simulink model "Outer_Tensor_Stream_Ex1"  (R2025a)
settings: Solver=VariableStepAuto  StartTime=0.0  StopTime=1024  RelTol=1e-3
undefined symbols (not defined in the file): Correlation_ValidMode, DUT, L, vsva1596, xcvc1702
libraries: aieUtilities x8, aieDSP x1, vmcUtilities x1
settings Model: Creator=sdegala  LastModifiedBy=sdegala

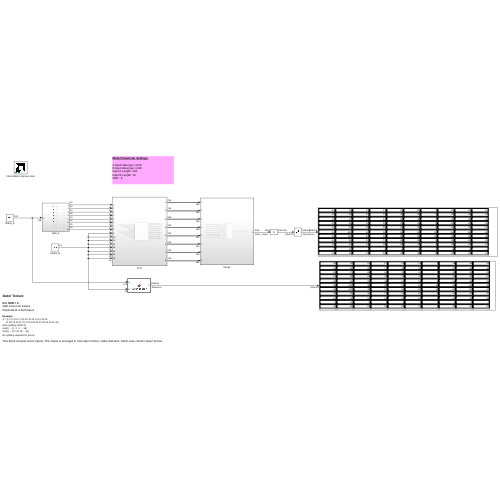
[thumbnail: Simulink's stored preview of the top-level diagram]
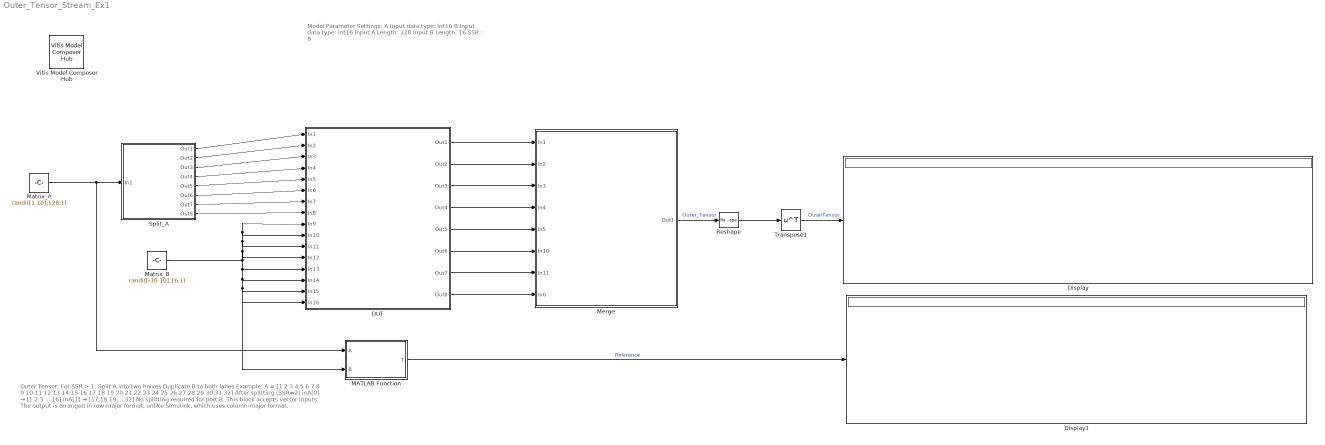
== system Outer_Tensor_Stream_Ex1 ==
  note: Model Parameter Settings:
      |
      | A Input data type: int16
      | B Input data type: int16
      | Input A Length: 128
      | Input B Length: 16
      | SSR : 8
  note: Outer Tensor:
      |
      | For SSR > 1:
      | Split A into two halves
      | Duplicate B to both lanes
      |
      | Example:
      | A = [1 2 3 4 5 6 7 8 9 10 11 12 13 14 15 16
      | 17 18 19 20 21 22 23 24 25 26 27 28 29 30 31 32]
      | After splitting (SSR=2)
      | inA[0] → [1 2 3 ... 16]
      | inA[1] → [17 18 19 ... 32]
      | No splitting required for port B.
      |
      | This block accepts vector inputs. The output is arranged in row-major format, unlike Simulink, which uses column-major format.
  DUT : Subsystem
  Display : Display
  Display1 : Display
  MATLAB Function : MATLAB Function  TreatAsAtomicUnit=on
  Matrix_A : Constant  Value=randi([1 10],128,1)  OutDataTypeStr=int16  SampleTime=1
  Matrix_B : Constant  Value=randi([-10 10],16,1)  OutDataTypeStr=int16  SampleTime=1
  Merge : Subsystem
  Reshape : Reshape  OutputDimensionality=Customize  OutputDimensions=[16,128]
  Split_A : Subsystem
  Transpose1 : Math  Operator=transpose
  Vitis Model Composer Hub : vmcUtilities/Vitis Model Composer Hub  Tag=genX  CodeGeneration=off  SubsystemName=DUT  BlockHierPath=Correlation_ValidMode/DUT  SubsystemType=AIENode  StartColumn=1  NumberOfColumns=1  TargetDirectory=./code  exportDesign=off  analyzeDesign=on  validateDesignOnHw=off  ExportType=AI Engines  IpVendor=xilinx.com  IpLibrary=hls  IpVersion=1.0  IpHWLanguage=Verilog  AieCompilerOptions={}  AieSimulatorOptions={}  CreateTestbench=on  TestbenchStackSize=10  RunRtlSim=off  RunCSim=off  RunAieSim=off  AieSimTimeout=50000  RunAieSimProfiling=off  LaunchVitisAnalyzer=off  PlotOutput=off  RunX86Sim=off  X86SimTimeout=10  GenHwImage=off  GenLibadfXo=off  GenHwValidationCode=off  PlatformType=Not Specified  HwSystemType=Baremetal  HwValidationTarget=hw  ProjDevice=xcvc1702-vsva1596-2LP-e-L  ProjDevicePart=xcvc1702-vsva1596-2LP-e-L  AIEType=AIE  SamplePeriod=-1  ClockFrequency=200  DataPathParallelism=1  xilinxfamily=versalaicore  part=xcvc1702  speed=-2LP-e-L  package=vsva1596  directory=./netlist  testbench=off  incr_netlist=off  synthesis_tool=Vivado  clock_wrapper=Clock Enables  dbl_ovrd=According to Block Masks  dcm_input_clock_period=10  sysclk_period=10  simulink_period=1  eval_field=0  IPInfoJsonString="{\"DUTSubsystemName\":\"DUT\",\"AIESubsystem\":{\"SubsystemName\":\"DUT\",\"TargetDirectory\":\"./code\",\"AIEArrayConfig\":\"Use entire AIE array\",\"StartColumn\":\"0\",\"NumberOfColumns\":\"1\"},\"SubsystemTag\":\"AIENode\"}"  LogFileName=/proj/xhdhdstaff5/sdegala/Head1/HEAD/2025_2_work/AIE_BLOCKS_2025_2/code/model_composer.log  NThreads=4  IPConfigFile=/tmp/vmctmp-11198269997411262707/Correlation_ValidMode_ipconfig.json
  wires:
  DUT/2(Out2) -> Merge/2(In2)
  Split_A/6(Out6) -> DUT/6(In6)
  Split_A/1(Out1) -> DUT/1(In1)
  Reshape/1 -> Transpose1/1
  DUT/1(Out1) -> Merge/1(In1)
  Split_A/8(Out8) -> DUT/8(In8)
  DUT/6(Out6) -> Merge/6(In10)
  Transpose1/1 -> Display/1  "OuterTensor"
  DUT/5(Out5) -> Merge/5(In5)
  DUT/8(Out8) -> Merge/8(In6)
  DUT/3(Out3) -> Merge/3(In3)
  MATLAB Function/1(T) -> Display1/1  "Reference"
  Matrix_A/1 -> MATLAB Function/1(A), Split_A/1(In1)
  Split_A/5(Out5) -> DUT/5(In5)
  Split_A/2(Out2) -> DUT/2(In2)
  DUT/4(Out4) -> Merge/4(In4)
  Merge/1(Out1) -> Reshape/1  "Outer_Tensor"
  Split_A/4(Out4) -> DUT/4(In4)
  Split_A/3(Out3) -> DUT/3(In3)
  Matrix_B/1 -> DUT/14(In14), DUT/16(In16), MATLAB Function/2(B), DUT/15(In15), DUT/13(In13), DUT/9(In9), DUT/10(In10), DUT/11(In11), DUT/12(In12)
  DUT/7(Out7) -> Merge/7(In11)
  Split_A/7(Out7) -> DUT/7(In7)

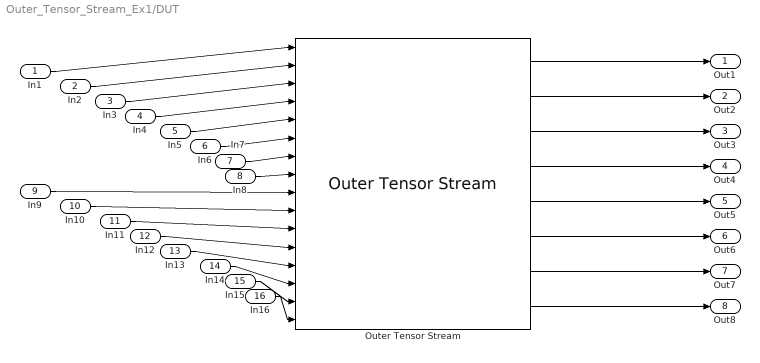
== system Outer_Tensor_Stream_Ex1/DUT ==
  In1 : Inport
  In2 : Inport  Port=2
  In3 : Inport  Port=3
  In4 : Inport  Port=4
  In5 : Inport  Port=5
  In6 : Inport  Port=6
  In7 : Inport  Port=7
  In8 : Inport  Port=8
  In9 : Inport  Port=9
  In10 : Inport  Port=10
  In11 : Inport  Port=11
  In12 : Inport  Port=12
  In13 : Inport  Port=13
  In14 : Inport  Port=14
  In15 : Inport  Port=15
  In16 : Inport  Port=16
  Outer Tensor Stream : aieDSP/Outer Tensor Stream  AIE_VARIANT=1  TP_API=1  data_type_A=int16  data_type_B=int16  dim_a=128  dim_b=16  num_frames=1  shift_output=0  ssr=8  rnd_mode=Floor  sat_mode=None  blockJsonConstraints=[]  blockJsonConstraintsInternal=[]  spec=vmc_stream_outer_tensor.json  SerializedMaskParamNames=[]  SerializedMaskParamValues=[]  SerializedMaskParamVisibilities=[]  block_type=Outer Tensor Stream  SerializedMaskParamDataypes=uint|uint|typename|typename|uint|uint|uint|uint|uint|uint|uint  SerializedMaskParamEnumStrArr=0|0|0|0|0|0|0|0|0|Floor,Ceiling,Round to positive infinity,Round to negative infinity,Round symmetrical to infinity,Round symmetrical to zero,Round convergent to even,Round convergent to odd|None,Saturate,Symmetric  SerializedMaskParamEnumValArr=0|0|0|0|0|0|0|0|0|0,1,2,3,4,5,6,7|0,1,3  SerializedMaskParamVectorArr=0|0|0|0|0|0|0|0|0|0|0  SerializedMaskParamKeys=AIE_VARIANT|TP_API|TT_DATA_A|TT_DATA_B|TP_DIM_A|TP_DIM_B|TP_NUM_FRAMES|TP_SHIFT|TP_SSR|TP_RND|TP_SAT
  Out1 : Outport
  Out2 : Outport  Port=2
  Out3 : Outport  Port=3
  Out4 : Outport  Port=4
  Out5 : Outport  Port=5
  Out6 : Outport  Port=6
  Out7 : Outport  Port=7
  Out8 : Outport  Port=8
  wires:
  In2/1 -> Outer Tensor Stream/2
  In1/1 -> Outer Tensor Stream/1
  Outer Tensor Stream/1 -> Out1/1
  In4/1 -> Outer Tensor Stream/4
  In3/1 -> Outer Tensor Stream/3
  Outer Tensor Stream/2 -> Out2/1
  In6/1 -> Outer Tensor Stream/6
  In5/1 -> Outer Tensor Stream/5
  In7/1 -> Outer Tensor Stream/7
  In8/1 -> Outer Tensor Stream/8
  In13/1 -> Outer Tensor Stream/13
  In12/1 -> Outer Tensor Stream/12
  In10/1 -> Outer Tensor Stream/10
  In11/1 -> Outer Tensor Stream/11
  In9/1 -> Outer Tensor Stream/9
  In14/1 -> Outer Tensor Stream/14
  In15/1 -> Outer Tensor Stream/15
  In16/1 -> Outer Tensor Stream/16
  Outer Tensor Stream/3 -> Out3/1
  Outer Tensor Stream/4 -> Out4/1
  Outer Tensor Stream/5 -> Out5/1
  Outer Tensor Stream/6 -> Out6/1
  Outer Tensor Stream/7 -> Out7/1
  Outer Tensor Stream/8 -> Out8/1

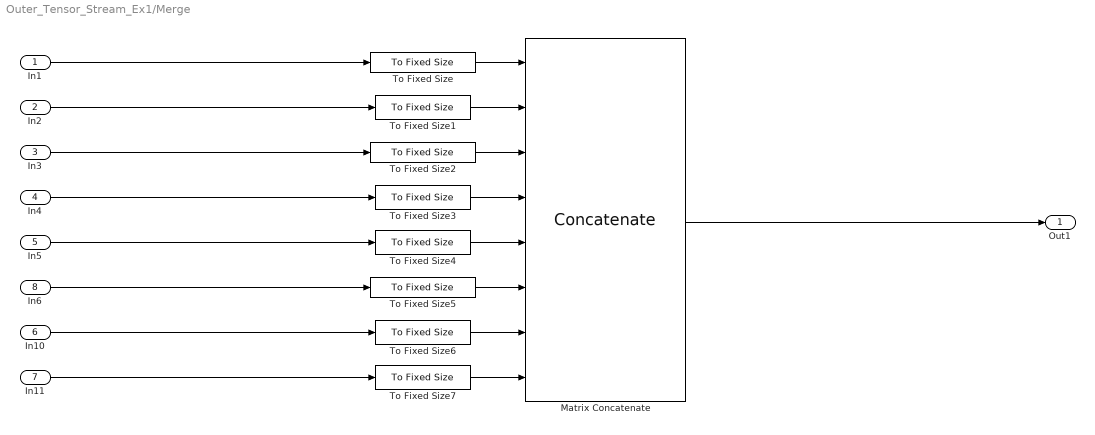
== system Outer_Tensor_Stream_Ex1/Merge ==
  In1 : Inport
  In2 : Inport  Port=2
  In3 : Inport  Port=3
  In4 : Inport  Port=4
  In5 : Inport  Port=5
  In10 : Inport  Port=6
  In11 : Inport  Port=7
  In6 : Inport  Port=8
  Matrix Concatenate : Concatenate  NumInputs=8  ConcatenateDimension=2
  To Fixed Size{,1..7} (8 alike) : aieUtilities/To Fixed Size  Mode=Stop simulation when input variable-size signal is not full  OutputSize=Inherit: Same as input  CopyMethod=Buffer samples to form output  HasStatusOutput=on
  Out1 : Outport
  wires:
  In1/1 -> To Fixed Size/1
  In2/1 -> To Fixed Size1/1
  To Fixed Size/1 -> Matrix Concatenate/1
  To Fixed Size1/1 -> Matrix Concatenate/2
  Matrix Concatenate/1 -> Out1/1
  In4/1 -> To Fixed Size3/1
  In3/1 -> To Fixed Size2/1
  To Fixed Size2/1 -> Matrix Concatenate/3
  To Fixed Size3/1 -> Matrix Concatenate/4
  To Fixed Size4/1 -> Matrix Concatenate/5
  In5/1 -> To Fixed Size4/1
  In6/1 -> To Fixed Size5/1
  In10/1 -> To Fixed Size6/1
  In11/1 -> To Fixed Size7/1
  To Fixed Size5/1 -> Matrix Concatenate/6
  To Fixed Size6/1 -> Matrix Concatenate/7
  To Fixed Size7/1 -> Matrix Concatenate/8

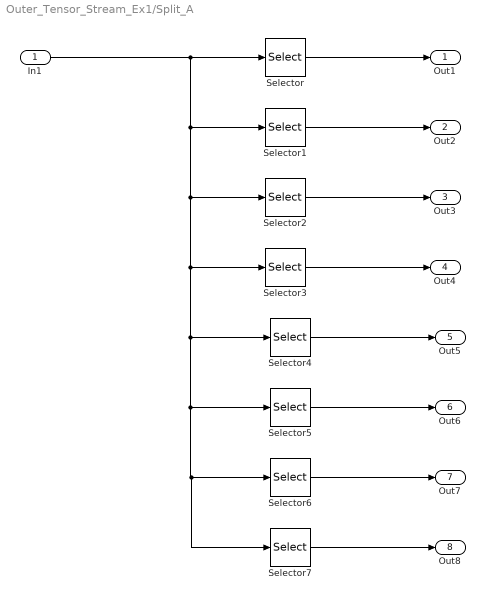
== system Outer_Tensor_Stream_Ex1/Split_A ==
  In1 : Inport
  Selector : Selector  InputPortWidth=128  IndexOptions=Index vector (dialog)  Indices=1:1:16  OutputSizes=1
  Selector1 : Selector  InputPortWidth=128  IndexOptions=Index vector (dialog)  Indices=17:1:32  OutputSizes=1
  Selector2 : Selector  InputPortWidth=128  IndexOptions=Index vector (dialog)  Indices=33:1:48  OutputSizes=1
  Selector3 : Selector  InputPortWidth=128  IndexOptions=Index vector (dialog)  Indices=49:1:64  OutputSizes=1
  Selector4 : Selector  InputPortWidth=128  IndexOptions=Index vector (dialog)  Indices=65:1:80  OutputSizes=1
  Selector5 : Selector  InputPortWidth=128  IndexOptions=Index vector (dialog)  Indices=81:1:96  OutputSizes=1
  Selector6 : Selector  InputPortWidth=128  IndexOptions=Index vector (dialog)  Indices=97:1:112  OutputSizes=1
  Selector7 : Selector  InputPortWidth=128  IndexOptions=Index vector (dialog)  Indices=113:1:128  OutputSizes=1
  Out1 : Outport
  Out2 : Outport  Port=2
  Out3 : Outport  Port=3
  Out4 : Outport  Port=4
  Out5 : Outport  Port=5
  Out6 : Outport  Port=6
  Out7 : Outport  Port=7
  Out8 : Outport  Port=8
  wires:
  Selector1/1 -> Out2/1
  Selector/1 -> Out1/1
  Selector2/1 -> Out3/1
  Selector3/1 -> Out4/1
  Selector7/1 -> Out8/1
  Selector5/1 -> Out6/1
  In1/1 -> Selector/1, Selector7/1, Selector6/1, Selector5/1, Selector4/1, Selector3/1, Selector2/1, Selector1/1
  Selector4/1 -> Out5/1
  Selector6/1 -> Out7/1

== matlab function Outer_Tensor_Stream_Ex1/MATLAB Function ==
  data: A input; T output; B input
function T = outer_tensor(A, B)
    szA = 128;
    szB = 16;

    Aexp = reshape(A, [szA ones(1,numel(szB))]);
    Bexp = reshape(B, [ones(1,numel(szA)) szB]);

    T = Aexp .* Bexp;
end
